simulink model "Open_scen_lucie_test_cs"  (R2019a)
settings: Solver=ode5  StartTime=0.0  StopTime=60  FixedStep=1/60  RelTol=1e-3
PreLoadFcn:
  | mbxruntime.callbacks.PreLoadFcn(bdroot);
PostLoadFcn:
  | mbxruntime.callbacks.PostLoadFcn(bdroot);
InitFcn:
  | mbxruntime.callbacks.InitFcn(bdroot);
StartFcn:
  | mbxruntime.callbacks.StartFcn(bdroot);
StopFcn:
  | mbxruntime.callbacks.StopFcn(bdroot);
model workspace: external: MAT-File .\Open_scen_lucie_test_cs_hws.mat (data not in the file)
undefined symbols (not defined in the file or in its folder): DiscIntNeverNeededParam, FovAzimuth, FovAzimuthDefined, FovElevation, FovElevationDefined, InitImageOutputDir, LocationX, LocationXDefined, LocationY, LocationYDefined, LocationZ, LocationZDefined, mbxruntime, Open_scen_lucie_test_cs_05b3fdca6ec99adc, Open_scen_lucie_test_cs_2d1bc0fbf6141b87, Open_scen_lucie_test_cs_453760b7ad36561d, Open_scen_lucie_test_cs_54de7300b247ce0d, Open_scen_lucie_test_cs_6819f386244a4b71, Open_scen_lucie_test_cs_685351e056f1bd0b, Open_scen_lucie_test_cs_6cd7f038842b0b77, Open_scen_lucie_test_cs_7a35ff65ce771bf6, Open_scen_lucie_test_cs_7ca083c9065fb1a1, Open_scen_lucie_test_cs_8bffacb258fa391b, Open_scen_lucie_test_cs_90e3bd399387ee5e, Open_scen_lucie_test_cs_a1176fb0c2e52fd1, Open_scen_lucie_test_cs_bb93306955583605, Open_scen_lucie_test_cs_c100ca66a180e443, Open_scen_lucie_test_cs_c1ddb1ec4c47a5f8, Open_scen_lucie_test_cs_ee3cfcef3d4d50fa, Open_scen_lucie_test_cs_f0142b471b498fb5, Open_scen_lucie_test_cs_fad1968c5de81336, OrientationPitch, OrientationPitchDefined, OrientationRoll, OrientationRollDefined, OrientationYaw, OrientationYawDefined, tabledata
libraries: adeye_lib x15, PreScanSimulinkLibrary x6, PreScanUsefulBlocks x1, simulink x1
(part 4 of 8)

== system Open_scen_lucie_test_cs/BMW_X5_SUV_1/CameraSensor_2_CM_Demux ==
  In1 : Inport
  Selector : Selector  NumberOfDimensions=2  InputPortWidth=3  IndexOptions=Index vector (dialog),Index vector (dialog)  Indices=-1,1:hres  OutputSizes=1,1
  Selector1 : Selector  NumberOfDimensions=2  InputPortWidth=3  IndexOptions=Index vector (dialog),Index vector (dialog)  Indices=-1,hres+1:hres*2  OutputSizes=1,1
  Selector2 : Selector  NumberOfDimensions=2  InputPortWidth=3  IndexOptions=Index vector (dialog),Index vector (dialog)  Indices=-1,hres*2+1:hres*3  OutputSizes=1,1
  R : Outport
  G : Outport  Port=2
  B : Outport  Port=3
  wires:
  In1/1 -> Selector1/1, Selector/1, Selector2/1
  Selector/1 -> R/1
  Selector1/1 -> G/1
  Selector2/1 -> B/1

== system Open_scen_lucie_test_cs/BMW_X5_SUV_1/CameraSensor_3_CM_Demux ==
  In1 : Inport
  Selector : Selector  NumberOfDimensions=2  InputPortWidth=3  IndexOptions=Index vector (dialog),Index vector (dialog)  Indices=-1,1:hres  OutputSizes=1,1
  Selector1 : Selector  NumberOfDimensions=2  InputPortWidth=3  IndexOptions=Index vector (dialog),Index vector (dialog)  Indices=-1,hres+1:hres*2  OutputSizes=1,1
  Selector2 : Selector  NumberOfDimensions=2  InputPortWidth=3  IndexOptions=Index vector (dialog),Index vector (dialog)  Indices=-1,hres*2+1:hres*3  OutputSizes=1,1
  R : Outport
  G : Outport  Port=2
  B : Outport  Port=3
  wires:
  In1/1 -> Selector1/1, Selector/1, Selector2/1
  Selector/1 -> R/1
  Selector1/1 -> G/1
  Selector2/1 -> B/1

== system Open_scen_lucie_test_cs/BMW_X5_SUV_1/CameraSensor_4_CM_Demux ==
  In1 : Inport
  Selector : Selector  NumberOfDimensions=2  InputPortWidth=3  IndexOptions=Index vector (dialog),Index vector (dialog)  Indices=-1,1:hres  OutputSizes=1,1
  Selector1 : Selector  NumberOfDimensions=2  InputPortWidth=3  IndexOptions=Index vector (dialog),Index vector (dialog)  Indices=-1,hres+1:hres*2  OutputSizes=1,1
  Selector2 : Selector  NumberOfDimensions=2  InputPortWidth=3  IndexOptions=Index vector (dialog),Index vector (dialog)  Indices=-1,hres*2+1:hres*3  OutputSizes=1,1
  R : Outport
  G : Outport  Port=2
  B : Outport  Port=3
  wires:
  In1/1 -> Selector1/1, Selector/1, Selector2/1
  Selector/1 -> R/1
  Selector1/1 -> G/1
  Selector2/1 -> B/1

== system Open_scen_lucie_test_cs/BMW_X5_SUV_1/Camera_1_CM_Demux ==
  In1 : Inport
  Selector : Selector  NumberOfDimensions=2  InputPortWidth=3  IndexOptions=Index vector (dialog),Index vector (dialog)  Indices=-1,1:hres  OutputSizes=1,1
  Selector1 : Selector  NumberOfDimensions=2  InputPortWidth=3  IndexOptions=Index vector (dialog),Index vector (dialog)  Indices=-1,hres+1:hres*2  OutputSizes=1,1
  Selector2 : Selector  NumberOfDimensions=2  InputPortWidth=3  IndexOptions=Index vector (dialog),Index vector (dialog)  Indices=-1,hres*2+1:hres*3  OutputSizes=1,1
  R : Outport
  G : Outport  Port=2
  B : Outport  Port=3
  wires:
  In1/1 -> Selector1/1, Selector/1, Selector2/1
  Selector/1 -> R/1
  Selector1/1 -> G/1
  Selector2/1 -> B/1

== system Open_scen_lucie_test_cs/BMW_X5_SUV_1/Camera_2_CM_Demux ==
  In1 : Inport
  Selector : Selector  NumberOfDimensions=2  InputPortWidth=3  IndexOptions=Index vector (dialog),Index vector (dialog)  Indices=-1,1:hres  OutputSizes=1,1
  Selector1 : Selector  NumberOfDimensions=2  InputPortWidth=3  IndexOptions=Index vector (dialog),Index vector (dialog)  Indices=-1,hres+1:hres*2  OutputSizes=1,1
  Selector2 : Selector  NumberOfDimensions=2  InputPortWidth=3  IndexOptions=Index vector (dialog),Index vector (dialog)  Indices=-1,hres*2+1:hres*3  OutputSizes=1,1
  R : Outport
  G : Outport  Port=2
  B : Outport  Port=3
  wires:
  In1/1 -> Selector1/1, Selector/1, Selector2/1
  Selector/1 -> R/1
  Selector1/1 -> G/1
  Selector2/1 -> B/1

== system Open_scen_lucie_test_cs/BMW_X5_SUV_1/Camera_tl_CM_Demux ==
  In1 : Inport
  Selector : Selector  NumberOfDimensions=2  InputPortWidth=3  IndexOptions=Index vector (dialog),Index vector (dialog)  Indices=-1,1:hres  OutputSizes=1,1
  Selector1 : Selector  NumberOfDimensions=2  InputPortWidth=3  IndexOptions=Index vector (dialog),Index vector (dialog)  Indices=-1,hres+1:hres*2  OutputSizes=1,1
  Selector2 : Selector  NumberOfDimensions=2  InputPortWidth=3  IndexOptions=Index vector (dialog),Index vector (dialog)  Indices=-1,hres*2+1:hres*3  OutputSizes=1,1
  R : Outport
  G : Outport  Port=2
  B : Outport  Port=3
  wires:
  In1/1 -> Selector1/1, Selector/1, Selector2/1
  Selector/1 -> R/1
  Selector1/1 -> G/1
  Selector2/1 -> B/1

== system Open_scen_lucie_test_cs/BMW_X5_SUV_1/Dynamics_Empty ==
  note: For state mode 'Dynamic' positions
      | are not taken into account, as they
      | are computed by integrating velocity.
      | Click annotation for Help.
  Ground_{1..9} (9 alike) : Ground
  MuxState : Subsystem  Tag=mux/State  mask(Empty Dynamics State Block){positioningmode=on, TimeStep=1/60}
      mask prompts: positioningmode "Positioning Mode"; TimeStep "Auto Assigned: Time Step [s]"
      mask help:
      | Build the state of an actor based on user input.
      | The user can either use positioning mode or dynamics mode.
      | - When using positioning mode the position and orientation of the actor are set directly based on the input. Expected input is relative to the initial position and orientation of the actor. It's also possible to specify the velocity of the actor, though this input isn't used, only passed on.
      | - When using dynamics mode the position input is ignored. Expected input is velocity and orientation. The velocity is relative the current orientation of the actor, while orientation is relative to its initial orientation. The position of the actor is calculated based on the velocity and orientation given.
      settings: DeleteFcn=PreScanBlockDeleteFcn;
  STATE_BMW_X5_SUV_1 : Subsystem  Tag=mux/StatePort  Priority=0  LoadFcn=load PrescanStateActuatorData  mask(PreScan Sink Block: State){x0=Open_scen_lucie_test_cs_c1ddb1ec4c47a5f8, y0=Open_scen_lucie_test_cs_05b3fdca6ec99adc, z0=Open_scen_lucie_test_cs_f0142b471b498fb5, Roll0=Open_scen_lucie_test_cs_a1176fb0c2e52fd1, Pitch0=Open_scen_lucie_test_cs_6cd7f038842b0b77, Yaw0=Open_scen_lucie_test_cs_90e3bd399387ee5e, TimeStep=1/60}
      mask prompts: x0 "Ini x-position VEHICLE wrt GLOBAL axis system [m]"; y0 "Ini y-position VEHICLE wrt GLOBAL axis system [m]"; z0 "Ini z-position VEHICLE wrt GLOBAL axis system [m]"; Roll0 "Ini roll-angle BODY wrt VEHICLE axis system [deg]"; Pitch0 "Ini pitch-angle BODY wrt VEHICLE axis system [deg]"; Yaw0 "Ini yaw-angle VEHICLE wrt GLOBAL axis system [deg]"; TimeStep "Auto-Assigned: Upload Period [s]"
      mask help:
      | The Actor State contains a vector signal of size (9x1), containing the following signals:
      |
      | -  Position                  (x,y,z)                                     [m]
      | -  Velocity                  (vx,vy,vz)                               [m/s]
      | -  Angles                    (Roll, Pitch, Yaw)                   [rad]
      |
      | The Actor state is defined in the global axis system.
      | The state is superponed on the Initial position defined in the GUI.
      |
      | For more information, please click Help.
      settings: DeleteFcn=PreScanBlockDeleteFcn;
      mask Help: eval('openHelp(222)')
      mask Display: image(imread('State.png'))
  State : Outport  Tag=outport/StateOutport  SampleTime=1/60
  wires:
  MuxState/1(state) -> STATE_BMW_X5_SUV_1/1(State)
  STATE_BMW_X5_SUV_1/1(StateBus) -> State/1
  Ground_1/1 -> MuxState/1(x [m])
  Ground_2/1 -> MuxState/2(y [m])
  Ground_3/1 -> MuxState/3(z [m])
  Ground_4/1 -> MuxState/4(dx [m/s])
  Ground_5/1 -> MuxState/5(dy [m/s])
  Ground_6/1 -> MuxState/6(dz [m/s])
  Ground_7/1 -> MuxState/7(R [rad])
  Ground_8/1 -> MuxState/8(P [rad])
  Ground_9/1 -> MuxState/9(Y [rad])

== system Open_scen_lucie_test_cs/BMW_X5_SUV_1/HumViewCamera_CM_Demux ==
  In1 : Inport
  Selector : Selector  NumberOfDimensions=2  InputPortWidth=3  IndexOptions=Index vector (dialog),Index vector (dialog)  Indices=-1,1:hres  OutputSizes=1,1
  Selector1 : Selector  NumberOfDimensions=2  InputPortWidth=3  IndexOptions=Index vector (dialog),Index vector (dialog)  Indices=-1,hres+1:hres*2  OutputSizes=1,1
  Selector2 : Selector  NumberOfDimensions=2  InputPortWidth=3  IndexOptions=Index vector (dialog),Index vector (dialog)  Indices=-1,hres*2+1:hres*3  OutputSizes=1,1
  R : Outport
  G : Outport  Port=2
  B : Outport  Port=3
  wires:
  In1/1 -> Selector1/1, Selector/1, Selector2/1
  Selector/1 -> R/1
  Selector1/1 -> G/1
  Selector2/1 -> B/1

== system Open_scen_lucie_test_cs/BMW_X5_SUV_1/Mux_CameraSensor_2_TA ==
  Location : Inport  Tag=inport/Camera_TA  OutDataTypeStr=double  PortDimensions=3  BusOutputAsStruct=on
  Orientation : Inport  Tag=inport/Camera_TA  Port=2  OutDataTypeStr=double  PortDimensions=3  BusOutputAsStruct=on
  IntensityFactorRGBMono : Inport  Tag=inport/Camera_TA  Port=3  OutDataTypeStr=double  PortDimensions=3  BusOutputAsStruct=on
  FoVAzimuth : Inport  Tag=inport/Camera_TA  Port=4  OutDataTypeStr=double  PortDimensions=1  BusOutputAsStruct=on
  FoVElevation : Inport  Tag=inport/Camera_TA  Port=5  OutDataTypeStr=double  PortDimensions=1  BusOutputAsStruct=on
  MisAlignMountPos : Inport  Tag=inport/Camera_TA  Port=6  OutDataTypeStr=double  PortDimensions=3  BusOutputAsStruct=on
  MisAlignMountOrient : Inport  Tag=inport/Camera_TA  Port=7  OutDataTypeStr=double  PortDimensions=3  BusOutputAsStruct=on
  Bus Assignment TA : BusAssignment  AssignedSignals=LocationX,LocationY,LocationZ,OrientationRoll,OrientationPitch,OrientationYaw,IntensityFactorR,IntensityFactorG,IntensityFactorB,FoVAzimuth,FoVElevation,MisalignMountPosX,MisalignMountPosY,MisalignMountPosZ,MisalignMountOrientX,MisalignMountOrientY,MisalignMountOrientZ,LocationXDefined,LocationYDefined,LocationZDefined,OrientationRollDefined,OrientationPitchDefined,OrientationYawDefined,IntensityFactorRDefined,IntensityFactorGDefined,IntensityFactorBDefined,FoVAzimuthDefined,FoVElevationDefined,MisalignMountPosXDefined,MisalignMountPosYDefined,MisalignMountPosZDefined,MisalignMountOrientXDefined,MisalignMountOrientYDefined,MisalignMountOrientZDefined
  ENABLE : Constant  Tag=ENABLE  Value=true
  IntensityFactorRGBMono_vec : Demux  Outputs=3
  Location_vec : Demux  Outputs=3
  MisAlignMountOrient_vec : Demux  Outputs=3
  MisAlignMountPos_vec : Demux  Outputs=3
  Orientation_vec : Demux  Outputs=3
  TA_bus : Subsystem
  TA : Outport  Tag=outport/Camera_TA/CameraSensor  OutDataTypeStr=Bus: PRESCAN_CAMERASENSOR_TA  PortDimensions=1  SampleTime=1/60
  wires:
  Bus Assignment TA/1 -> TA/1
  Location/1 -> Location_vec/1
  Location_vec/1 -> Bus Assignment TA/2
  Location_vec/2 -> Bus Assignment TA/3
  Location_vec/3 -> Bus Assignment TA/4
  Orientation/1 -> Orientation_vec/1
  Orientation_vec/1 -> Bus Assignment TA/5
  Orientation_vec/2 -> Bus Assignment TA/6
  Orientation_vec/3 -> Bus Assignment TA/7
  IntensityFactorRGBMono/1 -> IntensityFactorRGBMono_vec/1
  IntensityFactorRGBMono_vec/1 -> Bus Assignment TA/8
  IntensityFactorRGBMono_vec/2 -> Bus Assignment TA/9
  IntensityFactorRGBMono_vec/3 -> Bus Assignment TA/10
  FoVAzimuth/1 -> Bus Assignment TA/11
  FoVElevation/1 -> Bus Assignment TA/12
  MisAlignMountPos/1 -> MisAlignMountPos_vec/1
  MisAlignMountPos_vec/1 -> Bus Assignment TA/13
  MisAlignMountPos_vec/2 -> Bus Assignment TA/14
  MisAlignMountPos_vec/3 -> Bus Assignment TA/15
  MisAlignMountOrient/1 -> MisAlignMountOrient_vec/1
  MisAlignMountOrient_vec/1 -> Bus Assignment TA/16
  MisAlignMountOrient_vec/2 -> Bus Assignment TA/17
  MisAlignMountOrient_vec/3 -> Bus Assignment TA/18
  ENABLE/1 -> Bus Assignment TA/19, Bus Assignment TA/20, Bus Assignment TA/21, Bus Assignment TA/22, Bus Assignment TA/23, Bus Assignment TA/24, Bus Assignment TA/25, Bus Assignment TA/26, Bus Assignment TA/27, Bus Assignment TA/28, Bus Assignment TA/29, Bus Assignment TA/30, Bus Assignment TA/31, Bus Assignment TA/32, Bus Assignment TA/33, Bus Assignment TA/34, Bus Assignment TA/35
  TA_bus/1(bus) -> Bus Assignment TA/1

== system Open_scen_lucie_test_cs/BMW_X5_SUV_1/Mux_CameraSensor_3_TA ==
  Location : Inport  Tag=inport/Camera_TA  OutDataTypeStr=double  PortDimensions=3  BusOutputAsStruct=on
  Orientation : Inport  Tag=inport/Camera_TA  Port=2  OutDataTypeStr=double  PortDimensions=3  BusOutputAsStruct=on
  IntensityFactorRGBMono : Inport  Tag=inport/Camera_TA  Port=3  OutDataTypeStr=double  PortDimensions=3  BusOutputAsStruct=on
  FoVAzimuth : Inport  Tag=inport/Camera_TA  Port=4  OutDataTypeStr=double  PortDimensions=1  BusOutputAsStruct=on
  FoVElevation : Inport  Tag=inport/Camera_TA  Port=5  OutDataTypeStr=double  PortDimensions=1  BusOutputAsStruct=on
  MisAlignMountPos : Inport  Tag=inport/Camera_TA  Port=6  OutDataTypeStr=double  PortDimensions=3  BusOutputAsStruct=on
  MisAlignMountOrient : Inport  Tag=inport/Camera_TA  Port=7  OutDataTypeStr=double  PortDimensions=3  BusOutputAsStruct=on
  Bus Assignment TA : BusAssignment  AssignedSignals=LocationX,LocationY,LocationZ,OrientationRoll,OrientationPitch,OrientationYaw,IntensityFactorR,IntensityFactorG,IntensityFactorB,FoVAzimuth,FoVElevation,MisalignMountPosX,MisalignMountPosY,MisalignMountPosZ,MisalignMountOrientX,MisalignMountOrientY,MisalignMountOrientZ,LocationXDefined,LocationYDefined,LocationZDefined,OrientationRollDefined,OrientationPitchDefined,OrientationYawDefined,IntensityFactorRDefined,IntensityFactorGDefined,IntensityFactorBDefined,FoVAzimuthDefined,FoVElevationDefined,MisalignMountPosXDefined,MisalignMountPosYDefined,MisalignMountPosZDefined,MisalignMountOrientXDefined,MisalignMountOrientYDefined,MisalignMountOrientZDefined
  ENABLE : Constant  Tag=ENABLE  Value=true
  IntensityFactorRGBMono_vec : Demux  Outputs=3
  Location_vec : Demux  Outputs=3
  MisAlignMountOrient_vec : Demux  Outputs=3
  MisAlignMountPos_vec : Demux  Outputs=3
  Orientation_vec : Demux  Outputs=3
  TA_bus : Subsystem
  TA : Outport  Tag=outport/Camera_TA/CameraSensor  OutDataTypeStr=Bus: PRESCAN_CAMERASENSOR_TA  PortDimensions=1  SampleTime=1/60
  wires:
  Bus Assignment TA/1 -> TA/1
  Location/1 -> Location_vec/1
  Location_vec/1 -> Bus Assignment TA/2
  Location_vec/2 -> Bus Assignment TA/3
  Location_vec/3 -> Bus Assignment TA/4
  Orientation/1 -> Orientation_vec/1
  Orientation_vec/1 -> Bus Assignment TA/5
  Orientation_vec/2 -> Bus Assignment TA/6
  Orientation_vec/3 -> Bus Assignment TA/7
  IntensityFactorRGBMono/1 -> IntensityFactorRGBMono_vec/1
  IntensityFactorRGBMono_vec/1 -> Bus Assignment TA/8
  IntensityFactorRGBMono_vec/2 -> Bus Assignment TA/9
  IntensityFactorRGBMono_vec/3 -> Bus Assignment TA/10
  FoVAzimuth/1 -> Bus Assignment TA/11
  FoVElevation/1 -> Bus Assignment TA/12
  MisAlignMountPos/1 -> MisAlignMountPos_vec/1
  MisAlignMountPos_vec/1 -> Bus Assignment TA/13
  MisAlignMountPos_vec/2 -> Bus Assignment TA/14
  MisAlignMountPos_vec/3 -> Bus Assignment TA/15
  MisAlignMountOrient/1 -> MisAlignMountOrient_vec/1
  MisAlignMountOrient_vec/1 -> Bus Assignment TA/16
  MisAlignMountOrient_vec/2 -> Bus Assignment TA/17
  MisAlignMountOrient_vec/3 -> Bus Assignment TA/18
  ENABLE/1 -> Bus Assignment TA/19, Bus Assignment TA/20, Bus Assignment TA/21, Bus Assignment TA/22, Bus Assignment TA/23, Bus Assignment TA/24, Bus Assignment TA/25, Bus Assignment TA/26, Bus Assignment TA/27, Bus Assignment TA/28, Bus Assignment TA/29, Bus Assignment TA/30, Bus Assignment TA/31, Bus Assignment TA/32, Bus Assignment TA/33, Bus Assignment TA/34, Bus Assignment TA/35
  TA_bus/1(bus) -> Bus Assignment TA/1

== system Open_scen_lucie_test_cs/BMW_X5_SUV_1/Mux_CameraSensor_4_TA ==
  Location : Inport  Tag=inport/Camera_TA  OutDataTypeStr=double  PortDimensions=3  BusOutputAsStruct=on
  Orientation : Inport  Tag=inport/Camera_TA  Port=2  OutDataTypeStr=double  PortDimensions=3  BusOutputAsStruct=on
  IntensityFactorRGBMono : Inport  Tag=inport/Camera_TA  Port=3  OutDataTypeStr=double  PortDimensions=3  BusOutputAsStruct=on
  FoVAzimuth : Inport  Tag=inport/Camera_TA  Port=4  OutDataTypeStr=double  PortDimensions=1  BusOutputAsStruct=on
  FoVElevation : Inport  Tag=inport/Camera_TA  Port=5  OutDataTypeStr=double  PortDimensions=1  BusOutputAsStruct=on
  MisAlignMountPos : Inport  Tag=inport/Camera_TA  Port=6  OutDataTypeStr=double  PortDimensions=3  BusOutputAsStruct=on
  MisAlignMountOrient : Inport  Tag=inport/Camera_TA  Port=7  OutDataTypeStr=double  PortDimensions=3  BusOutputAsStruct=on
  Bus Assignment TA : BusAssignment  AssignedSignals=LocationX,LocationY,LocationZ,OrientationRoll,OrientationPitch,OrientationYaw,IntensityFactorR,IntensityFactorG,IntensityFactorB,FoVAzimuth,FoVElevation,MisalignMountPosX,MisalignMountPosY,MisalignMountPosZ,MisalignMountOrientX,MisalignMountOrientY,MisalignMountOrientZ,LocationXDefined,LocationYDefined,LocationZDefined,OrientationRollDefined,OrientationPitchDefined,OrientationYawDefined,IntensityFactorRDefined,IntensityFactorGDefined,IntensityFactorBDefined,FoVAzimuthDefined,FoVElevationDefined,MisalignMountPosXDefined,MisalignMountPosYDefined,MisalignMountPosZDefined,MisalignMountOrientXDefined,MisalignMountOrientYDefined,MisalignMountOrientZDefined
  ENABLE : Constant  Tag=ENABLE  Value=true
  IntensityFactorRGBMono_vec : Demux  Outputs=3
  Location_vec : Demux  Outputs=3
  MisAlignMountOrient_vec : Demux  Outputs=3
  MisAlignMountPos_vec : Demux  Outputs=3
  Orientation_vec : Demux  Outputs=3
  TA_bus : Subsystem
  TA : Outport  Tag=outport/Camera_TA/CameraSensor  OutDataTypeStr=Bus: PRESCAN_CAMERASENSOR_TA  PortDimensions=1  SampleTime=1/60
  wires:
  Bus Assignment TA/1 -> TA/1
  Location/1 -> Location_vec/1
  Location_vec/1 -> Bus Assignment TA/2
  Location_vec/2 -> Bus Assignment TA/3
  Location_vec/3 -> Bus Assignment TA/4
  Orientation/1 -> Orientation_vec/1
  Orientation_vec/1 -> Bus Assignment TA/5
  Orientation_vec/2 -> Bus Assignment TA/6
  Orientation_vec/3 -> Bus Assignment TA/7
  IntensityFactorRGBMono/1 -> IntensityFactorRGBMono_vec/1
  IntensityFactorRGBMono_vec/1 -> Bus Assignment TA/8
  IntensityFactorRGBMono_vec/2 -> Bus Assignment TA/9
  IntensityFactorRGBMono_vec/3 -> Bus Assignment TA/10
  FoVAzimuth/1 -> Bus Assignment TA/11
  FoVElevation/1 -> Bus Assignment TA/12
  MisAlignMountPos/1 -> MisAlignMountPos_vec/1
  MisAlignMountPos_vec/1 -> Bus Assignment TA/13
  MisAlignMountPos_vec/2 -> Bus Assignment TA/14
  MisAlignMountPos_vec/3 -> Bus Assignment TA/15
  MisAlignMountOrient/1 -> MisAlignMountOrient_vec/1
  MisAlignMountOrient_vec/1 -> Bus Assignment TA/16
  MisAlignMountOrient_vec/2 -> Bus Assignment TA/17
  MisAlignMountOrient_vec/3 -> Bus Assignment TA/18
  ENABLE/1 -> Bus Assignment TA/19, Bus Assignment TA/20, Bus Assignment TA/21, Bus Assignment TA/22, Bus Assignment TA/23, Bus Assignment TA/24, Bus Assignment TA/25, Bus Assignment TA/26, Bus Assignment TA/27, Bus Assignment TA/28, Bus Assignment TA/29, Bus Assignment TA/30, Bus Assignment TA/31, Bus Assignment TA/32, Bus Assignment TA/33, Bus Assignment TA/34, Bus Assignment TA/35
  TA_bus/1(bus) -> Bus Assignment TA/1

== system Open_scen_lucie_test_cs/BMW_X5_SUV_1/Mux_Camera_1_TA ==
  Location : Inport  Tag=inport/Camera_TA  OutDataTypeStr=double  PortDimensions=3  BusOutputAsStruct=on
  Orientation : Inport  Tag=inport/Camera_TA  Port=2  OutDataTypeStr=double  PortDimensions=3  BusOutputAsStruct=on
  IntensityFactorRGBMono : Inport  Tag=inport/Camera_TA  Port=3  OutDataTypeStr=double  PortDimensions=3  BusOutputAsStruct=on
  FoVAzimuth : Inport  Tag=inport/Camera_TA  Port=4  OutDataTypeStr=double  PortDimensions=1  BusOutputAsStruct=on
  FoVElevation : Inport  Tag=inport/Camera_TA  Port=5  OutDataTypeStr=double  PortDimensions=1  BusOutputAsStruct=on
  MisAlignMountPos : Inport  Tag=inport/Camera_TA  Port=6  OutDataTypeStr=double  PortDimensions=3  BusOutputAsStruct=on
  MisAlignMountOrient : Inport  Tag=inport/Camera_TA  Port=7  OutDataTypeStr=double  PortDimensions=3  BusOutputAsStruct=on
  Bus Assignment TA : BusAssignment  AssignedSignals=LocationX,LocationY,LocationZ,OrientationRoll,OrientationPitch,OrientationYaw,IntensityFactorR,IntensityFactorG,IntensityFactorB,FoVAzimuth,FoVElevation,MisalignMountPosX,MisalignMountPosY,MisalignMountPosZ,MisalignMountOrientX,MisalignMountOrientY,MisalignMountOrientZ,LocationXDefined,LocationYDefined,LocationZDefined,OrientationRollDefined,OrientationPitchDefined,OrientationYawDefined,IntensityFactorRDefined,IntensityFactorGDefined,IntensityFactorBDefined,FoVAzimuthDefined,FoVElevationDefined,MisalignMountPosXDefined,MisalignMountPosYDefined,MisalignMountPosZDefined,MisalignMountOrientXDefined,MisalignMountOrientYDefined,MisalignMountOrientZDefined
  ENABLE : Constant  Tag=ENABLE  Value=true
  IntensityFactorRGBMono_vec : Demux  Outputs=3
  Location_vec : Demux  Outputs=3
  MisAlignMountOrient_vec : Demux  Outputs=3
  MisAlignMountPos_vec : Demux  Outputs=3
  Orientation_vec : Demux  Outputs=3
  TA_bus : Subsystem
  TA : Outport  Tag=outport/Camera_TA/CameraSensor  OutDataTypeStr=Bus: PRESCAN_CAMERASENSOR_TA  PortDimensions=1  SampleTime=1/60
  wires:
  Bus Assignment TA/1 -> TA/1
  Location/1 -> Location_vec/1
  Location_vec/1 -> Bus Assignment TA/2
  Location_vec/2 -> Bus Assignment TA/3
  Location_vec/3 -> Bus Assignment TA/4
  Orientation/1 -> Orientation_vec/1
  Orientation_vec/1 -> Bus Assignment TA/5
  Orientation_vec/2 -> Bus Assignment TA/6
  Orientation_vec/3 -> Bus Assignment TA/7
  IntensityFactorRGBMono/1 -> IntensityFactorRGBMono_vec/1
  IntensityFactorRGBMono_vec/1 -> Bus Assignment TA/8
  IntensityFactorRGBMono_vec/2 -> Bus Assignment TA/9
  IntensityFactorRGBMono_vec/3 -> Bus Assignment TA/10
  FoVAzimuth/1 -> Bus Assignment TA/11
  FoVElevation/1 -> Bus Assignment TA/12
  MisAlignMountPos/1 -> MisAlignMountPos_vec/1
  MisAlignMountPos_vec/1 -> Bus Assignment TA/13
  MisAlignMountPos_vec/2 -> Bus Assignment TA/14
  MisAlignMountPos_vec/3 -> Bus Assignment TA/15
  MisAlignMountOrient/1 -> MisAlignMountOrient_vec/1
  MisAlignMountOrient_vec/1 -> Bus Assignment TA/16
  MisAlignMountOrient_vec/2 -> Bus Assignment TA/17
  MisAlignMountOrient_vec/3 -> Bus Assignment TA/18
  ENABLE/1 -> Bus Assignment TA/19, Bus Assignment TA/20, Bus Assignment TA/21, Bus Assignment TA/22, Bus Assignment TA/23, Bus Assignment TA/24, Bus Assignment TA/25, Bus Assignment TA/26, Bus Assignment TA/27, Bus Assignment TA/28, Bus Assignment TA/29, Bus Assignment TA/30, Bus Assignment TA/31, Bus Assignment TA/32, Bus Assignment TA/33, Bus Assignment TA/34, Bus Assignment TA/35
  TA_bus/1(bus) -> Bus Assignment TA/1

== system Open_scen_lucie_test_cs/BMW_X5_SUV_1/Mux_Camera_2_TA ==
  Location : Inport  Tag=inport/Camera_TA  OutDataTypeStr=double  PortDimensions=3  BusOutputAsStruct=on
  Orientation : Inport  Tag=inport/Camera_TA  Port=2  OutDataTypeStr=double  PortDimensions=3  BusOutputAsStruct=on
  IntensityFactorRGBMono : Inport  Tag=inport/Camera_TA  Port=3  OutDataTypeStr=double  PortDimensions=3  BusOutputAsStruct=on
  FoVAzimuth : Inport  Tag=inport/Camera_TA  Port=4  OutDataTypeStr=double  PortDimensions=1  BusOutputAsStruct=on
  FoVElevation : Inport  Tag=inport/Camera_TA  Port=5  OutDataTypeStr=double  PortDimensions=1  BusOutputAsStruct=on
  MisAlignMountPos : Inport  Tag=inport/Camera_TA  Port=6  OutDataTypeStr=double  PortDimensions=3  BusOutputAsStruct=on
  MisAlignMountOrient : Inport  Tag=inport/Camera_TA  Port=7  OutDataTypeStr=double  PortDimensions=3  BusOutputAsStruct=on
  Bus Assignment TA : BusAssignment  AssignedSignals=LocationX,LocationY,LocationZ,OrientationRoll,OrientationPitch,OrientationYaw,IntensityFactorR,IntensityFactorG,IntensityFactorB,FoVAzimuth,FoVElevation,MisalignMountPosX,MisalignMountPosY,MisalignMountPosZ,MisalignMountOrientX,MisalignMountOrientY,MisalignMountOrientZ,LocationXDefined,LocationYDefined,LocationZDefined,OrientationRollDefined,OrientationPitchDefined,OrientationYawDefined,IntensityFactorRDefined,IntensityFactorGDefined,IntensityFactorBDefined,FoVAzimuthDefined,FoVElevationDefined,MisalignMountPosXDefined,MisalignMountPosYDefined,MisalignMountPosZDefined,MisalignMountOrientXDefined,MisalignMountOrientYDefined,MisalignMountOrientZDefined
  ENABLE : Constant  Tag=ENABLE  Value=true
  IntensityFactorRGBMono_vec : Demux  Outputs=3
  Location_vec : Demux  Outputs=3
  MisAlignMountOrient_vec : Demux  Outputs=3
  MisAlignMountPos_vec : Demux  Outputs=3
  Orientation_vec : Demux  Outputs=3
  TA_bus : Subsystem
  TA : Outport  Tag=outport/Camera_TA/CameraSensor  OutDataTypeStr=Bus: PRESCAN_CAMERASENSOR_TA  PortDimensions=1  SampleTime=1/60
  wires:
  Bus Assignment TA/1 -> TA/1
  Location/1 -> Location_vec/1
  Location_vec/1 -> Bus Assignment TA/2
  Location_vec/2 -> Bus Assignment TA/3
  Location_vec/3 -> Bus Assignment TA/4
  Orientation/1 -> Orientation_vec/1
  Orientation_vec/1 -> Bus Assignment TA/5
  Orientation_vec/2 -> Bus Assignment TA/6
  Orientation_vec/3 -> Bus Assignment TA/7
  IntensityFactorRGBMono/1 -> IntensityFactorRGBMono_vec/1
  IntensityFactorRGBMono_vec/1 -> Bus Assignment TA/8
  IntensityFactorRGBMono_vec/2 -> Bus Assignment TA/9
  IntensityFactorRGBMono_vec/3 -> Bus Assignment TA/10
  FoVAzimuth/1 -> Bus Assignment TA/11
  FoVElevation/1 -> Bus Assignment TA/12
  MisAlignMountPos/1 -> MisAlignMountPos_vec/1
  MisAlignMountPos_vec/1 -> Bus Assignment TA/13
  MisAlignMountPos_vec/2 -> Bus Assignment TA/14
  MisAlignMountPos_vec/3 -> Bus Assignment TA/15
  MisAlignMountOrient/1 -> MisAlignMountOrient_vec/1
  MisAlignMountOrient_vec/1 -> Bus Assignment TA/16
  MisAlignMountOrient_vec/2 -> Bus Assignment TA/17
  MisAlignMountOrient_vec/3 -> Bus Assignment TA/18
  ENABLE/1 -> Bus Assignment TA/19, Bus Assignment TA/20, Bus Assignment TA/21, Bus Assignment TA/22, Bus Assignment TA/23, Bus Assignment TA/24, Bus Assignment TA/25, Bus Assignment TA/26, Bus Assignment TA/27, Bus Assignment TA/28, Bus Assignment TA/29, Bus Assignment TA/30, Bus Assignment TA/31, Bus Assignment TA/32, Bus Assignment TA/33, Bus Assignment TA/34, Bus Assignment TA/35
  TA_bus/1(bus) -> Bus Assignment TA/1

== system Open_scen_lucie_test_cs/BMW_X5_SUV_1/Mux_Camera_tl_TA ==
  Location : Inport  Tag=inport/Camera_TA  OutDataTypeStr=double  PortDimensions=3  BusOutputAsStruct=on
  Orientation : Inport  Tag=inport/Camera_TA  Port=2  OutDataTypeStr=double  PortDimensions=3  BusOutputAsStruct=on
  IntensityFactorRGBMono : Inport  Tag=inport/Camera_TA  Port=3  OutDataTypeStr=double  PortDimensions=3  BusOutputAsStruct=on
  FoVAzimuth : Inport  Tag=inport/Camera_TA  Port=4  OutDataTypeStr=double  PortDimensions=1  BusOutputAsStruct=on
  FoVElevation : Inport  Tag=inport/Camera_TA  Port=5  OutDataTypeStr=double  PortDimensions=1  BusOutputAsStruct=on
  MisAlignMountPos : Inport  Tag=inport/Camera_TA  Port=6  OutDataTypeStr=double  PortDimensions=3  BusOutputAsStruct=on
  MisAlignMountOrient : Inport  Tag=inport/Camera_TA  Port=7  OutDataTypeStr=double  PortDimensions=3  BusOutputAsStruct=on
  Bus Assignment TA : BusAssignment  AssignedSignals=LocationX,LocationY,LocationZ,OrientationRoll,OrientationPitch,OrientationYaw,IntensityFactorR,IntensityFactorG,IntensityFactorB,FoVAzimuth,FoVElevation,MisalignMountPosX,MisalignMountPosY,MisalignMountPosZ,MisalignMountOrientX,MisalignMountOrientY,MisalignMountOrientZ,LocationXDefined,LocationYDefined,LocationZDefined,OrientationRollDefined,OrientationPitchDefined,OrientationYawDefined,IntensityFactorRDefined,IntensityFactorGDefined,IntensityFactorBDefined,FoVAzimuthDefined,FoVElevationDefined,MisalignMountPosXDefined,MisalignMountPosYDefined,MisalignMountPosZDefined,MisalignMountOrientXDefined,MisalignMountOrientYDefined,MisalignMountOrientZDefined
  ENABLE : Constant  Tag=ENABLE  Value=true
  IntensityFactorRGBMono_vec : Demux  Outputs=3
  Location_vec : Demux  Outputs=3
  MisAlignMountOrient_vec : Demux  Outputs=3
  MisAlignMountPos_vec : Demux  Outputs=3
  Orientation_vec : Demux  Outputs=3
  TA_bus : Subsystem
  TA : Outport  Tag=outport/Camera_TA/CameraSensor  OutDataTypeStr=Bus: PRESCAN_CAMERASENSOR_TA  PortDimensions=1  SampleTime=1/60
  wires:
  Bus Assignment TA/1 -> TA/1
  Location/1 -> Location_vec/1
  Location_vec/1 -> Bus Assignment TA/2
  Location_vec/2 -> Bus Assignment TA/3
  Location_vec/3 -> Bus Assignment TA/4
  Orientation/1 -> Orientation_vec/1
  Orientation_vec/1 -> Bus Assignment TA/5
  Orientation_vec/2 -> Bus Assignment TA/6
  Orientation_vec/3 -> Bus Assignment TA/7
  IntensityFactorRGBMono/1 -> IntensityFactorRGBMono_vec/1
  IntensityFactorRGBMono_vec/1 -> Bus Assignment TA/8
  IntensityFactorRGBMono_vec/2 -> Bus Assignment TA/9
  IntensityFactorRGBMono_vec/3 -> Bus Assignment TA/10
  FoVAzimuth/1 -> Bus Assignment TA/11
  FoVElevation/1 -> Bus Assignment TA/12
  MisAlignMountPos/1 -> MisAlignMountPos_vec/1
  MisAlignMountPos_vec/1 -> Bus Assignment TA/13
  MisAlignMountPos_vec/2 -> Bus Assignment TA/14
  MisAlignMountPos_vec/3 -> Bus Assignment TA/15
  MisAlignMountOrient/1 -> MisAlignMountOrient_vec/1
  MisAlignMountOrient_vec/1 -> Bus Assignment TA/16
  MisAlignMountOrient_vec/2 -> Bus Assignment TA/17
  MisAlignMountOrient_vec/3 -> Bus Assignment TA/18
  ENABLE/1 -> Bus Assignment TA/19, Bus Assignment TA/20, Bus Assignment TA/21, Bus Assignment TA/22, Bus Assignment TA/23, Bus Assignment TA/24, Bus Assignment TA/25, Bus Assignment TA/26, Bus Assignment TA/27, Bus Assignment TA/28, Bus Assignment TA/29, Bus Assignment TA/30, Bus Assignment TA/31, Bus Assignment TA/32, Bus Assignment TA/33, Bus Assignment TA/34, Bus Assignment TA/35
  TA_bus/1(bus) -> Bus Assignment TA/1

== system Open_scen_lucie_test_cs/BMW_X5_SUV_1/Mux_HumViewCamera_TA ==
  Location : Inport  Tag=inport/Camera_TA  OutDataTypeStr=double  PortDimensions=3  BusOutputAsStruct=on
  Orientation : Inport  Tag=inport/Camera_TA  Port=2  OutDataTypeStr=double  PortDimensions=3  BusOutputAsStruct=on
  IntensityFactorRGBMono : Inport  Tag=inport/Camera_TA  Port=3  OutDataTypeStr=double  PortDimensions=3  BusOutputAsStruct=on
  FoVAzimuth : Inport  Tag=inport/Camera_TA  Port=4  OutDataTypeStr=double  PortDimensions=1  BusOutputAsStruct=on
  FoVElevation : Inport  Tag=inport/Camera_TA  Port=5  OutDataTypeStr=double  PortDimensions=1  BusOutputAsStruct=on
  MisAlignMountPos : Inport  Tag=inport/Camera_TA  Port=6  OutDataTypeStr=double  PortDimensions=3  BusOutputAsStruct=on
  MisAlignMountOrient : Inport  Tag=inport/Camera_TA  Port=7  OutDataTypeStr=double  PortDimensions=3  BusOutputAsStruct=on
  Bus Assignment TA : BusAssignment  AssignedSignals=LocationX,LocationY,LocationZ,OrientationRoll,OrientationPitch,OrientationYaw,IntensityFactorR,IntensityFactorG,IntensityFactorB,FoVAzimuth,FoVElevation,MisalignMountPosX,MisalignMountPosY,MisalignMountPosZ,MisalignMountOrientX,MisalignMountOrientY,MisalignMountOrientZ,LocationXDefined,LocationYDefined,LocationZDefined,OrientationRollDefined,OrientationPitchDefined,OrientationYawDefined,IntensityFactorRDefined,IntensityFactorGDefined,IntensityFactorBDefined,FoVAzimuthDefined,FoVElevationDefined,MisalignMountPosXDefined,MisalignMountPosYDefined,MisalignMountPosZDefined,MisalignMountOrientXDefined,MisalignMountOrientYDefined,MisalignMountOrientZDefined
  ENABLE : Constant  Tag=ENABLE  Value=true
  IntensityFactorRGBMono_vec : Demux  Outputs=3
  Location_vec : Demux  Outputs=3
  MisAlignMountOrient_vec : Demux  Outputs=3
  MisAlignMountPos_vec : Demux  Outputs=3
  Orientation_vec : Demux  Outputs=3
  TA_bus : Subsystem
  TA : Outport  Tag=outport/Camera_TA/CameraSensor  OutDataTypeStr=Bus: PRESCAN_CAMERASENSOR_TA  PortDimensions=1  SampleTime=1/60
  wires:
  Bus Assignment TA/1 -> TA/1
  Location/1 -> Location_vec/1
  Location_vec/1 -> Bus Assignment TA/2
  Location_vec/2 -> Bus Assignment TA/3
  Location_vec/3 -> Bus Assignment TA/4
  Orientation/1 -> Orientation_vec/1
  Orientation_vec/1 -> Bus Assignment TA/5
  Orientation_vec/2 -> Bus Assignment TA/6
  Orientation_vec/3 -> Bus Assignment TA/7
  IntensityFactorRGBMono/1 -> IntensityFactorRGBMono_vec/1
  IntensityFactorRGBMono_vec/1 -> Bus Assignment TA/8
  IntensityFactorRGBMono_vec/2 -> Bus Assignment TA/9
  IntensityFactorRGBMono_vec/3 -> Bus Assignment TA/10
  FoVAzimuth/1 -> Bus Assignment TA/11
  FoVElevation/1 -> Bus Assignment TA/12
  MisAlignMountPos/1 -> MisAlignMountPos_vec/1
  MisAlignMountPos_vec/1 -> Bus Assignment TA/13
  MisAlignMountPos_vec/2 -> Bus Assignment TA/14
  MisAlignMountPos_vec/3 -> Bus Assignment TA/15
  MisAlignMountOrient/1 -> MisAlignMountOrient_vec/1
  MisAlignMountOrient_vec/1 -> Bus Assignment TA/16
  MisAlignMountOrient_vec/2 -> Bus Assignment TA/17
  MisAlignMountOrient_vec/3 -> Bus Assignment TA/18
  ENABLE/1 -> Bus Assignment TA/19, Bus Assignment TA/20, Bus Assignment TA/21, Bus Assignment TA/22, Bus Assignment TA/23, Bus Assignment TA/24, Bus Assignment TA/25, Bus Assignment TA/26, Bus Assignment TA/27, Bus Assignment TA/28, Bus Assignment TA/29, Bus Assignment TA/30, Bus Assignment TA/31, Bus Assignment TA/32, Bus Assignment TA/33, Bus Assignment TA/34, Bus Assignment TA/35
  TA_bus/1(bus) -> Bus Assignment TA/1

== system Open_scen_lucie_test_cs/BMW_X5_SUV_1/Mux_PointCloudSensor_1_TA ==
  Location : Inport  Tag=inport/PointCloud_TA  OutDataTypeStr=double  PortDimensions=3  BusOutputAsStruct=on
  Orientation : Inport  Tag=inport/PointCloud_TA  Port=2  OutDataTypeStr=double  PortDimensions=3  BusOutputAsStruct=on
  FovAzimuth : Inport  Tag=inport/PointCloud_TA  Port=3  OutDataTypeStr=double  PortDimensions=1  BusOutputAsStruct=on
  FovElevation : Inport  Tag=inport/PointCloud_TA  Port=4  OutDataTypeStr=double  PortDimensions=1  BusOutputAsStruct=on
  Bus Assignment TA : BusAssignment  AssignedSignals=LocationX,LocationY,LocationZ,OrientationRoll,OrientationPitch,OrientationYaw,FovAzimuth,FovElevation,LocationXDefined,LocationYDefined,LocationZDefined,OrientationRollDefined,OrientationPitchDefined,OrientationYawDefined,FovAzimuthDefined,FovElevationDefined
  ENABLE : Constant  Tag=ENABLE  Value=true
  Location_vec : Demux  Outputs=3
  Orientation_vec : Demux  Outputs=3
  TA_bus : Subsystem
  TA : Outport  Tag=outport/SensorTA  OutDataTypeStr=Bus: PRESCAN_PCS_TA_DATA  PortDimensions=1  SampleTime=1/60
  wires:
  Bus Assignment TA/1 -> TA/1
  Location/1 -> Location_vec/1
  Location_vec/1 -> Bus Assignment TA/2
  Location_vec/2 -> Bus Assignment TA/3
  Location_vec/3 -> Bus Assignment TA/4
  Orientation/1 -> Orientation_vec/1
  Orientation_vec/1 -> Bus Assignment TA/5
  Orientation_vec/2 -> Bus Assignment TA/6
  Orientation_vec/3 -> Bus Assignment TA/7
  FovAzimuth/1 -> Bus Assignment TA/8
  FovElevation/1 -> Bus Assignment TA/9
  ENABLE/1 -> Bus Assignment TA/10, Bus Assignment TA/11, Bus Assignment TA/12, Bus Assignment TA/13, Bus Assignment TA/14, Bus Assignment TA/15, Bus Assignment TA/16, Bus Assignment TA/17
  TA_bus/1(bus) -> Bus Assignment TA/1

== system Open_scen_lucie_test_cs/BMW_X5_SUV_1/Mux_PointCloudSensor_2_TA ==
  Location : Inport  Tag=inport/PointCloud_TA  OutDataTypeStr=double  PortDimensions=3  BusOutputAsStruct=on
  Orientation : Inport  Tag=inport/PointCloud_TA  Port=2  OutDataTypeStr=double  PortDimensions=3  BusOutputAsStruct=on
  FovAzimuth : Inport  Tag=inport/PointCloud_TA  Port=3  OutDataTypeStr=double  PortDimensions=1  BusOutputAsStruct=on
  FovElevation : Inport  Tag=inport/PointCloud_TA  Port=4  OutDataTypeStr=double  PortDimensions=1  BusOutputAsStruct=on
  Bus Assignment TA : BusAssignment  AssignedSignals=LocationX,LocationY,LocationZ,OrientationRoll,OrientationPitch,OrientationYaw,FovAzimuth,FovElevation,LocationXDefined,LocationYDefined,LocationZDefined,OrientationRollDefined,OrientationPitchDefined,OrientationYawDefined,FovAzimuthDefined,FovElevationDefined
  ENABLE : Constant  Tag=ENABLE  Value=true
  Location_vec : Demux  Outputs=3
  Orientation_vec : Demux  Outputs=3
  TA_bus : Subsystem
  TA : Outport  Tag=outport/SensorTA  OutDataTypeStr=Bus: PRESCAN_PCS_TA_DATA  PortDimensions=1  SampleTime=1/60
  wires:
  Bus Assignment TA/1 -> TA/1
  Location/1 -> Location_vec/1
  Location_vec/1 -> Bus Assignment TA/2
  Location_vec/2 -> Bus Assignment TA/3
  Location_vec/3 -> Bus Assignment TA/4
  Orientation/1 -> Orientation_vec/1
  Orientation_vec/1 -> Bus Assignment TA/5
  Orientation_vec/2 -> Bus Assignment TA/6
  Orientation_vec/3 -> Bus Assignment TA/7
  FovAzimuth/1 -> Bus Assignment TA/8
  FovElevation/1 -> Bus Assignment TA/9
  ENABLE/1 -> Bus Assignment TA/10, Bus Assignment TA/11, Bus Assignment TA/12, Bus Assignment TA/13, Bus Assignment TA/14, Bus Assignment TA/15, Bus Assignment TA/16, Bus Assignment TA/17
  TA_bus/1(bus) -> Bus Assignment TA/1

== system Open_scen_lucie_test_cs/BMW_X5_SUV_1/Mux_PointCloudSensor_3_TA ==
  Location : Inport  Tag=inport/PointCloud_TA  OutDataTypeStr=double  PortDimensions=3  BusOutputAsStruct=on
  Orientation : Inport  Tag=inport/PointCloud_TA  Port=2  OutDataTypeStr=double  PortDimensions=3  BusOutputAsStruct=on
  FovAzimuth : Inport  Tag=inport/PointCloud_TA  Port=3  OutDataTypeStr=double  PortDimensions=1  BusOutputAsStruct=on
  FovElevation : Inport  Tag=inport/PointCloud_TA  Port=4  OutDataTypeStr=double  PortDimensions=1  BusOutputAsStruct=on
  Bus Assignment TA : BusAssignment  AssignedSignals=LocationX,LocationY,LocationZ,OrientationRoll,OrientationPitch,OrientationYaw,FovAzimuth,FovElevation,LocationXDefined,LocationYDefined,LocationZDefined,OrientationRollDefined,OrientationPitchDefined,OrientationYawDefined,FovAzimuthDefined,FovElevationDefined
  ENABLE : Constant  Tag=ENABLE  Value=true
  Location_vec : Demux  Outputs=3
  Orientation_vec : Demux  Outputs=3
  TA_bus : Subsystem
  TA : Outport  Tag=outport/SensorTA  OutDataTypeStr=Bus: PRESCAN_PCS_TA_DATA  PortDimensions=1  SampleTime=1/60
  wires:
  Bus Assignment TA/1 -> TA/1
  Location/1 -> Location_vec/1
  Location_vec/1 -> Bus Assignment TA/2
  Location_vec/2 -> Bus Assignment TA/3
  Location_vec/3 -> Bus Assignment TA/4
  Orientation/1 -> Orientation_vec/1
  Orientation_vec/1 -> Bus Assignment TA/5
  Orientation_vec/2 -> Bus Assignment TA/6
  Orientation_vec/3 -> Bus Assignment TA/7
  FovAzimuth/1 -> Bus Assignment TA/8
  FovElevation/1 -> Bus Assignment TA/9
  ENABLE/1 -> Bus Assignment TA/10, Bus Assignment TA/11, Bus Assignment TA/12, Bus Assignment TA/13, Bus Assignment TA/14, Bus Assignment TA/15, Bus Assignment TA/16, Bus Assignment TA/17
  TA_bus/1(bus) -> Bus Assignment TA/1

== system Open_scen_lucie_test_cs/BMW_X5_SUV_1/Mux_PointCloudSensor_4_TA ==
  Location : Inport  Tag=inport/PointCloud_TA  OutDataTypeStr=double  PortDimensions=3  BusOutputAsStruct=on
  Orientation : Inport  Tag=inport/PointCloud_TA  Port=2  OutDataTypeStr=double  PortDimensions=3  BusOutputAsStruct=on
  FovAzimuth : Inport  Tag=inport/PointCloud_TA  Port=3  OutDataTypeStr=double  PortDimensions=1  BusOutputAsStruct=on
  FovElevation : Inport  Tag=inport/PointCloud_TA  Port=4  OutDataTypeStr=double  PortDimensions=1  BusOutputAsStruct=on
  Bus Assignment TA : BusAssignment  AssignedSignals=LocationX,LocationY,LocationZ,OrientationRoll,OrientationPitch,OrientationYaw,FovAzimuth,FovElevation,LocationXDefined,LocationYDefined,LocationZDefined,OrientationRollDefined,OrientationPitchDefined,OrientationYawDefined,FovAzimuthDefined,FovElevationDefined
  ENABLE : Constant  Tag=ENABLE  Value=true
  Location_vec : Demux  Outputs=3
  Orientation_vec : Demux  Outputs=3
  TA_bus : Subsystem
  TA : Outport  Tag=outport/SensorTA  OutDataTypeStr=Bus: PRESCAN_PCS_TA_DATA  PortDimensions=1  SampleTime=1/60
  wires:
  Bus Assignment TA/1 -> TA/1
  Location/1 -> Location_vec/1
  Location_vec/1 -> Bus Assignment TA/2
  Location_vec/2 -> Bus Assignment TA/3
  Location_vec/3 -> Bus Assignment TA/4
  Orientation/1 -> Orientation_vec/1
  Orientation_vec/1 -> Bus Assignment TA/5
  Orientation_vec/2 -> Bus Assignment TA/6
  Orientation_vec/3 -> Bus Assignment TA/7
  FovAzimuth/1 -> Bus Assignment TA/8
  FovElevation/1 -> Bus Assignment TA/9
  ENABLE/1 -> Bus Assignment TA/10, Bus Assignment TA/11, Bus Assignment TA/12, Bus Assignment TA/13, Bus Assignment TA/14, Bus Assignment TA/15, Bus Assignment TA/16, Bus Assignment TA/17
  TA_bus/1(bus) -> Bus Assignment TA/1

== system Open_scen_lucie_test_cs/BMW_X5_SUV_1/Mux_Radar_1_TA ==
  Location : Inport  Tag=inport/Radar_TA  OutDataTypeStr=double  PortDimensions=3  BusOutputAsStruct=on
  Orientation : Inport  Tag=inport/Radar_TA  Port=2  OutDataTypeStr=double  PortDimensions=3  BusOutputAsStruct=on
  Range : Inport  Tag=inport/Radar_TA  Port=3  OutDataTypeStr=double  PortDimensions=1  BusOutputAsStruct=on
  NoiseAzimuthIllumination : Inport  Tag=inport/Radar_TA  Port=4  OutDataTypeStr=double  PortDimensions=1  BusOutputAsStruct=on
  NoiseAziIlluType : Inport  Tag=inport/Radar_TA  Port=5  OutDataTypeStr=uint32  PortDimensions=1  BusOutputAsStruct=on
  NoiseElevationIllumination : Inport  Tag=inport/Radar_TA  Port=6  OutDataTypeStr=double  PortDimensions=1  BusOutputAsStruct=on
  NoiseElevIlluType : Inport  Tag=inport/Radar_TA  Port=7  OutDataTypeStr=uint32  PortDimensions=1  BusOutputAsStruct=on
  NoiseAzimuthReflection : Inport  Tag=inport/Radar_TA  Port=8  OutDataTypeStr=double  PortDimensions=1  BusOutputAsStruct=on
  NoiseAziReflectType : Inport  Tag=inport/Radar_TA  Port=9  OutDataTypeStr=uint32  PortDimensions=1  BusOutputAsStruct=on
  NoiseElevationReflection : Inport  Tag=inport/Radar_TA  Port=10  OutDataTypeStr=double  PortDimensions=1  BusOutputAsStruct=on
  NoiseElevReflectType : Inport  Tag=inport/Radar_TA  Port=11  OutDataTypeStr=uint32  PortDimensions=1  BusOutputAsStruct=on
  NoiseRange : Inport  Tag=inport/Radar_TA  Port=12  OutDataTypeStr=double  PortDimensions=1  BusOutputAsStruct=on
  NoiseRangeType : Inport  Tag=inport/Radar_TA  Port=13  OutDataTypeStr=uint32  PortDimensions=1  BusOutputAsStruct=on
  Bus Assignment TA : BusAssignment  AssignedSignals=LocationX,LocationY,LocationZ,OrientationRoll,OrientationPitch,OrientationYaw,Range,NoiseAzimuthIllumination,NoiseAziIlluType,NoiseElevationIllumination,NoiseElevIlluType,NoiseAzimuthReflection,NoiseAziReflectType,NoiseElevationReflection,NoiseElevReflectType,NoiseRange,NoiseRangeType,LocationXDefined,LocationYDefined,LocationZDefined,OrientationRollDefined,OrientationPitchDefined,OrientationYawDefined,RangeDefined,NoiseAzimuthIlluminationDefined,NoiseAziIlluTypeDefined,NoiseElevationIlluminationDefined,NoiseElevIlluTypeDefined,NoiseAzimuthReflectionDefined,NoiseAziReflectTypeDefined,NoiseElevationReflectionDefined,NoiseElevReflectTypeDefined,NoiseRangeDefined,NoiseRangeTypeDefined
  ENABLE : Constant  Tag=ENABLE  Value=true
  Location_vec : Demux  Outputs=3
  Orientation_vec : Demux  Outputs=3
  TA_bus : Subsystem
  TA : Outport  Tag=outport/Radar_TA  OutDataTypeStr=Bus: PRESCAN_SCANNERSENSOR_TA  PortDimensions=1  SampleTime=1/60
  wires:
  Bus Assignment TA/1 -> TA/1
  Location/1 -> Location_vec/1
  Location_vec/1 -> Bus Assignment TA/2
  Location_vec/2 -> Bus Assignment TA/3
  Location_vec/3 -> Bus Assignment TA/4
  Orientation/1 -> Orientation_vec/1
  Orientation_vec/1 -> Bus Assignment TA/5
  Orientation_vec/2 -> Bus Assignment TA/6
  Orientation_vec/3 -> Bus Assignment TA/7
  Range/1 -> Bus Assignment TA/8
  NoiseAzimuthIllumination/1 -> Bus Assignment TA/9
  NoiseAziIlluType/1 -> Bus Assignment TA/10
  NoiseElevationIllumination/1 -> Bus Assignment TA/11
  NoiseElevIlluType/1 -> Bus Assignment TA/12
  NoiseAzimuthReflection/1 -> Bus Assignment TA/13
  NoiseAziReflectType/1 -> Bus Assignment TA/14
  NoiseElevationReflection/1 -> Bus Assignment TA/15
  NoiseElevReflectType/1 -> Bus Assignment TA/16
  NoiseRange/1 -> Bus Assignment TA/17
  NoiseRangeType/1 -> Bus Assignment TA/18
  ENABLE/1 -> Bus Assignment TA/19, Bus Assignment TA/20, Bus Assignment TA/21, Bus Assignment TA/22, Bus Assignment TA/23, Bus Assignment TA/24, Bus Assignment TA/25, Bus Assignment TA/26, Bus Assignment TA/27, Bus Assignment TA/28, Bus Assignment TA/29, Bus Assignment TA/30, Bus Assignment TA/31, Bus Assignment TA/32, Bus Assignment TA/33, Bus Assignment TA/34, Bus Assignment TA/35
  TA_bus/1(bus) -> Bus Assignment TA/1

== system Open_scen_lucie_test_cs/BMW_X5_SUV_1/PointCloudSensor_1_Angles_Demux ==
  In2 : Inport
  Selector : Selector  NumberOfDimensions=2  InputPortWidth=3  IndexOptions=Index vector (dialog),Index vector (dialog)  Indices=-1,offset+1:(offset+hres)  OutputSizes=1,1
  Selector1 : Selector  NumberOfDimensions=2  InputPortWidth=3  IndexOptions=Index vector (dialog),Index vector (dialog)  Indices=-1,(offset+hres+1):(offset+2*hres)  OutputSizes=1,1
  Theta : Outport
  Phi : Outport  Port=2
  wires:
  Selector1/1 -> Phi/1
  Selector/1 -> Theta/1
  In2/1 -> Selector/1, Selector1/1

== system Open_scen_lucie_test_cs/BMW_X5_SUV_1/PointCloudSensor_1_Intensity_Demux ==
  In1 : Inport
  Selector3 : Selector  NumberOfDimensions=2  InputPortWidth=3  IndexOptions=Index vector (dialog),Index vector (dialog)  Indices=-1,offset+1:(offset+hres)  OutputSizes=1,1
  Intensity : Outport
  wires:
  Selector3/1 -> Intensity/1
  In1/1 -> Selector3/1

== system Open_scen_lucie_test_cs/BMW_X5_SUV_1/PointCloudSensor_1_Range_Demux ==
  In1 : Inport
  Selector : Selector  NumberOfDimensions=2  InputPortWidth=3  IndexOptions=Index vector (dialog),Index vector (dialog)  Indices=-1,offset+1:(offset+hres)  OutputSizes=1,1
  Range : Outport
  wires:
  Selector/1 -> Range/1
  In1/1 -> Selector/1

== system Open_scen_lucie_test_cs/BMW_X5_SUV_1/PointCloudSensor_2_Angles_Demux ==
  In2 : Inport
  Selector : Selector  NumberOfDimensions=2  InputPortWidth=3  IndexOptions=Index vector (dialog),Index vector (dialog)  Indices=-1,offset+1:(offset+hres)  OutputSizes=1,1
  Selector1 : Selector  NumberOfDimensions=2  InputPortWidth=3  IndexOptions=Index vector (dialog),Index vector (dialog)  Indices=-1,(offset+hres+1):(offset+2*hres)  OutputSizes=1,1
  Theta : Outport
  Phi : Outport  Port=2
  wires:
  Selector1/1 -> Phi/1
  Selector/1 -> Theta/1
  In2/1 -> Selector/1, Selector1/1

== system Open_scen_lucie_test_cs/BMW_X5_SUV_1/PointCloudSensor_2_Intensity_Demux ==
  In1 : Inport
  Selector3 : Selector  NumberOfDimensions=2  InputPortWidth=3  IndexOptions=Index vector (dialog),Index vector (dialog)  Indices=-1,offset+1:(offset+hres)  OutputSizes=1,1
  Intensity : Outport
  wires:
  Selector3/1 -> Intensity/1
  In1/1 -> Selector3/1

== system Open_scen_lucie_test_cs/BMW_X5_SUV_1/PointCloudSensor_2_Range_Demux ==
  In1 : Inport
  Selector : Selector  NumberOfDimensions=2  InputPortWidth=3  IndexOptions=Index vector (dialog),Index vector (dialog)  Indices=-1,offset+1:(offset+hres)  OutputSizes=1,1
  Range : Outport
  wires:
  Selector/1 -> Range/1
  In1/1 -> Selector/1

== system Open_scen_lucie_test_cs/BMW_X5_SUV_1/PointCloudSensor_3_Angles_Demux ==
  In2 : Inport
  Selector : Selector  NumberOfDimensions=2  InputPortWidth=3  IndexOptions=Index vector (dialog),Index vector (dialog)  Indices=-1,offset+1:(offset+hres)  OutputSizes=1,1
  Selector1 : Selector  NumberOfDimensions=2  InputPortWidth=3  IndexOptions=Index vector (dialog),Index vector (dialog)  Indices=-1,(offset+hres+1):(offset+2*hres)  OutputSizes=1,1
  Theta : Outport
  Phi : Outport  Port=2
  wires:
  Selector1/1 -> Phi/1
  Selector/1 -> Theta/1
  In2/1 -> Selector/1, Selector1/1

== system Open_scen_lucie_test_cs/BMW_X5_SUV_1/PointCloudSensor_3_Intensity_Demux ==
  In1 : Inport
  Selector3 : Selector  NumberOfDimensions=2  InputPortWidth=3  IndexOptions=Index vector (dialog),Index vector (dialog)  Indices=-1,offset+1:(offset+hres)  OutputSizes=1,1
  Intensity : Outport
  wires:
  Selector3/1 -> Intensity/1
  In1/1 -> Selector3/1

== system Open_scen_lucie_test_cs/BMW_X5_SUV_1/PointCloudSensor_3_Range_Demux ==
  In1 : Inport
  Selector : Selector  NumberOfDimensions=2  InputPortWidth=3  IndexOptions=Index vector (dialog),Index vector (dialog)  Indices=-1,offset+1:(offset+hres)  OutputSizes=1,1
  Range : Outport
  wires:
  Selector/1 -> Range/1
  In1/1 -> Selector/1

== system Open_scen_lucie_test_cs/BMW_X5_SUV_1/PointCloudSensor_4_Angles_Demux ==
  In2 : Inport
  Selector : Selector  NumberOfDimensions=2  InputPortWidth=3  IndexOptions=Index vector (dialog),Index vector (dialog)  Indices=-1,offset+1:(offset+hres)  OutputSizes=1,1
  Selector1 : Selector  NumberOfDimensions=2  InputPortWidth=3  IndexOptions=Index vector (dialog),Index vector (dialog)  Indices=-1,(offset+hres+1):(offset+2*hres)  OutputSizes=1,1
  Theta : Outport
  Phi : Outport  Port=2
  wires:
  Selector1/1 -> Phi/1
  Selector/1 -> Theta/1
  In2/1 -> Selector/1, Selector1/1

== system Open_scen_lucie_test_cs/BMW_X5_SUV_1/PointCloudSensor_4_Intensity_Demux ==
  In1 : Inport
  Selector3 : Selector  NumberOfDimensions=2  InputPortWidth=3  IndexOptions=Index vector (dialog),Index vector (dialog)  Indices=-1,offset+1:(offset+hres)  OutputSizes=1,1
  Intensity : Outport
  wires:
  Selector3/1 -> Intensity/1
  In1/1 -> Selector3/1

== system Open_scen_lucie_test_cs/BMW_X5_SUV_1/PointCloudSensor_4_Range_Demux ==
  In1 : Inport
  Selector : Selector  NumberOfDimensions=2  InputPortWidth=3  IndexOptions=Index vector (dialog),Index vector (dialog)  Indices=-1,offset+1:(offset+hres)  OutputSizes=1,1
  Range : Outport
  wires:
  Selector/1 -> Range/1
  In1/1 -> Selector/1

== system Open_scen_lucie_test_cs/BMW_X5_SUV_1/Radar_1_Demux ==
  Radar : Inport
  Bus Selector1 : BusSelector  OutputSignals=ActiveBeamID[-],Range[m],DopplerVelocity[ms-1],DopplerVelocityX[ms-1],DopplerVelocityY[ms-1],DopplerVelocityZ[ms-1],Theta[deg],Phi[deg],TargetID[-],TargetTypeID[-],EnergyLoss[dB],Alpha[deg],Beta[deg]  OutputAsBus=on
  ScannerSensorLegacyBusConversion : PreScanUsefulBlocks/ScannerSensorLegacyBusConversion  MAXMESSAGES=MAXMESSAGES
  Radar Data : Outport
  wires:
  Bus Selector1/1 -> Radar Data/1
  ScannerSensorLegacyBusConversion/1 -> Bus Selector1/1
  Radar/1 -> ScannerSensorLegacyBusConversion/1
